simulink model "example_WeatherDatafile_solar"  (R2018b)
settings: Solver=VariableStepAuto  StartTime=0.0  StopTime=365*24*3600  MaxStep=3600  RelTol=1e-3  EnableMultiTasking=on
undefined symbols (not defined in the file): path_carnot
libraries: carnot x2
settings Model: Creator=drhf  LastModifiedBy=drhf
settings DataIOCC: LimitDataPoints=on  SaveFormat=Array
settings OptimizationCC: ExpressionDepthLimit=2147483647  LifeSpan=inf
settings DebuggingCC: UnderspecifiedInitializationDetection=Classic  MergeDetectMultiDrivingBlocksExec=none  StateNameClashWarn=warning  SFUnexpectedBacktrackingDiag=warning  SFNoUnconditionalDefaultTransitionDiag=warning  SFExecutionAtInitializationDiag=none
settings HardwareCC: ProdBitPerPointer=32  ProdBitPerSizeT=32  ProdBitPerPtrDiffT=32  ProdLargestAtomicFloat=None  ProdIntDivRoundTo=Undefined  ProdEndianess=Unspecified  ProdWordSize=32  ProdHWDeviceType=32-bit Generic
settings ModelReferenceCC: PropagateSignalLabelsOutOfModel=off
settings SFSimCC: SimUseLocalCustomCode=off
settings RTWCC: RTWUseLocalCustomCode=off
settings CodeAppCC: StateflowObjectComments=on
settings GRTTargetCC: TargetLangStandard=C89/C90 (ANSI)  GeneratePreprocessorConditionals=Disable all  CombineOutputUpdateFcns=off  GRTInterface=on
settings ConfigComp: CovMetricSettings=dw  CovHtmlReporting=on  CovSaveCumulativeToWorkspaceVar=on  CovSaveSingleToWorkspaceVar=on  CovExternalEMLEnable=off

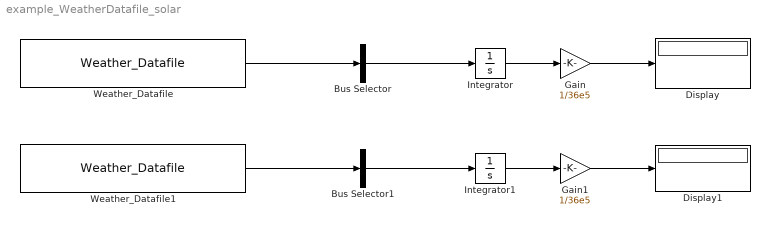
== system example_WeatherDatafile_solar ==
  Bus Selector : BusSelector  OutputSignals=Solar_Radiation_direct_surface,Solar_Radiation_diffuse_surface  OutputAsBus=on
  Bus Selector1 : BusSelector  OutputSignals=Solar_Radiation_direct_surface,Solar_Radiation_diffuse_surface  OutputAsBus=on
  Display : Display
  Display1 : Display
  Gain : Gain  Gain=1/36e5
  Gain1 : Gain  Gain=1/36e5
  Integrator : Integrator
  Integrator1 : Integrator
  Weather_Datafile : carnot/Weather/Weather_Datafile  PathName=path_carnot('data')  FileName='DE_TRY2010_04_averageYear.mat'  UserParam=off  VariableName=DE_TRY2010_01_extremeWinter  SampleTime=3600
      settings: SourceProductName=Carnot
  Weather_Datafile1 : carnot/Weather/Weather_Datafile  PathName=path_carnot('data')  FileName='DE_TRY2016_Potsdam_averageYear.mat'  UserParam=off  VariableName=DE_TRY2010_01_extremeWinter  SampleTime=3600
      settings: SourceProductName=Carnot
  wires:
  Weather_Datafile/1 -> Bus Selector/1
  Bus Selector/1 -> Integrator/1
  Weather_Datafile1/1 -> Bus Selector1/1
  Bus Selector1/1 -> Integrator1/1
  Integrator/1 -> Gain/1
  Integrator1/1 -> Gain1/1
  Gain/1 -> Display/1
  Gain1/1 -> Display1/1
